simulink model "example"  (R2015b)
settings: Solver=VariableStepAuto  StartTime=0.0  StopTime=10.0  RelTol=1e-3
undefined symbols (not defined in the file or in its folder): b
settings Model: Creator=mlish  LastModifiedBy=mlish
settings DataIOCC: LimitDataPoints=off

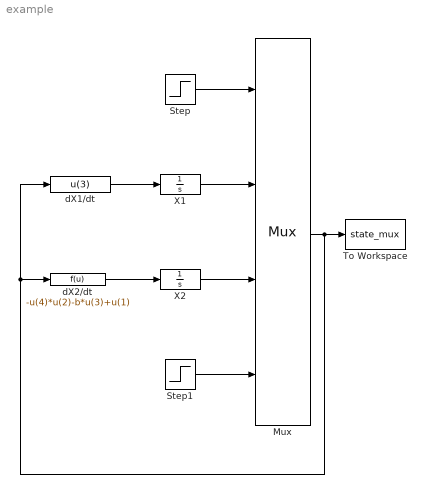
== system example ==
  Mux : Mux
      settings: DisplayOption=signals
  Step : Step  Time=0  SampleTime=0
  Step1 : Step  Time=5  Before=1  After=2  SampleTime=0
  To Workspace : ToWorkspace  VariableName=state_mux  SampleTime=-1
  X1 : Integrator
  X2 : Integrator
  dX1/dt : Fcn  Expr=u(3)
  dX2/dt : Fcn  Expr=-u(4)*u(2)-b*u(3)+u(1)
  wires:
  X1/1 -> Mux/2
  X2/1 -> Mux/3
  Step/1 -> Mux/1
  dX1/dt/1 -> X1/1
  dX2/dt/1 -> X2/1
  Mux/1 -> To Workspace/1, dX2/dt/1, dX1/dt/1
  Step1/1 -> Mux/4
